simulink model "GalvoModel_v3_tfCCneu_frd"  (R2013a)
settings: Solver=ode45  StartTime=0.0  StopTime=1.5  RelTol=1e-3
values from neighbouring files (symbols this model uses):
  BEM = 108e-6    (= 0.000108)    [GalvoModel_WOK_step.m]
  CL = 180e-6    (= 0.00018)    [GalvoModel_WOK_step.m]    (also in GalvoModel_v4_sys.m = @(x,n) repmat(x, 1, n); GalvoModel_v6_sys.m = @(x,n) repmat(x, 1, n))
  CR = 2.79    [GalvoModel_WOK_step.m]
  FR = 4e-12    [GalvoModel_WOK_step.m]
  H = 0.1403    [GalvoModel_v3_discret_proc.m]
  KTR = 47e-3    (= 0.047)    [GalvoModel_WOK_step.m]
  RIN = 1.25e-8    (= 1.25e-08)    [GalvoModel_WOK_step.m]
  TRC = 6.17e-3    (= 0.00617)    [GalvoModel_WOK_step.m]
libraries: cstblocks x1
settings Model: Creator=mainster  LastModifiedBy=mainster
settings DebuggingCC: SolverPrmCheckMsg=none

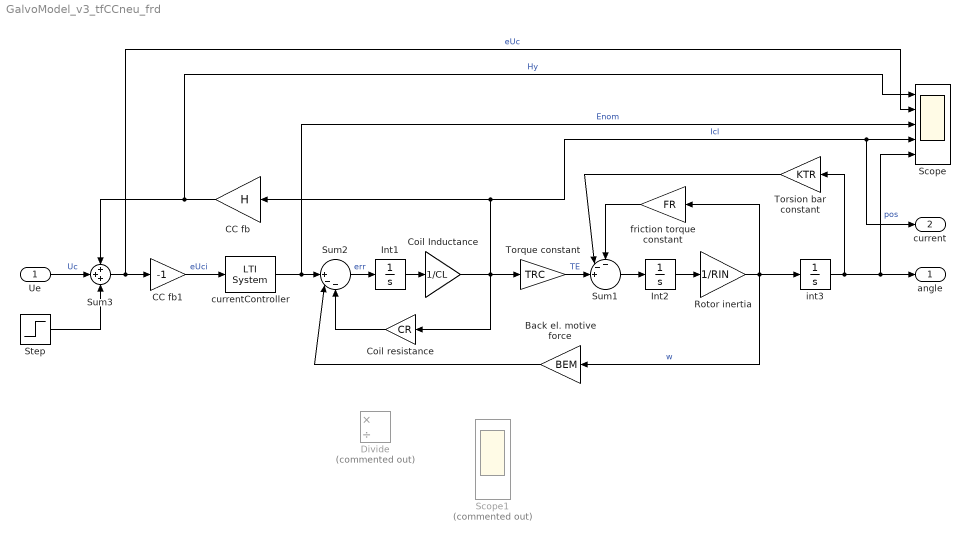
== system GalvoModel_v3_tfCCneu_frd ==
  Ue : Inport
  Back el. motive force : Gain  Gain=BEM
  CC fb : Gain  StartFcn=|  Gain=H
      | %H=100;                       
      | sprintf('StartFcn: H is %i',H)
      settings: AttributesFormatString=H=eval(%<Gain>)
  CC fb1 : Gain  StartFcn=|  Gain=-1
      | %H=100;                       
      | sprintf('StartFcn: H is %i',H)
  Coil Inductance : Gain  Gain=1/CL
  Coil resistance : Gain  Gain=CR
  Divide : Product  Commented=on  Inputs=*/
  Int1 : Integrator
  Int2 : Integrator
  Rotor inertia : Gain  Gain=1/RIN
  Scope : Scope  NumInputPorts=5
      settings: ShowLegends=on  TimeRange=1.5  YMin=-1~0.8~-15~-1~-0.2  YMax=1~1.05~5~4~1  MaxDataPoints=500000
  Scope1 : Scope  Commented=on  NumInputPorts=5
      settings: ShowLegends=on  TimeRange=1.5  YMin=-1~0.8~-15~-1~-0.2  YMax=1~1.05~5~4~1  MaxDataPoints=500000
  Step : Step  Time=0  SampleTime=0
  Sum1 : Sum  Inputs=--+||
  Sum2 : Sum  Inputs=||+--
  Sum3 : Sum  Inputs=+++
  Torque constant : Gain  Gain=TRC
  Torsion bar constant : Gain  Gain=KTR
  currentController : cstblocks/LTI System  sys=C  IC=[]
  friction torque constant : Gain  Gain=FR
  int3 : Integrator
  angle : Outport
  current : Outport  Port=2
  wires:
  Sum2/1 -> Int1/1  "err"
  Rotor inertia/1 -> Back el. motive force/1, int3/1, friction torque constant/1  "w"
  int3/1 -> Torsion bar constant/1, Scope/5, angle/1  "pos"
  Int1/1 -> Coil Inductance/1
  Coil resistance/1 -> Sum2/3
  Int2/1 -> Rotor inertia/1
  friction torque constant/1 -> Sum1/1
  Torsion bar constant/1 -> Sum1/2
  Torque constant/1 -> Sum1/3  "TE"
  Sum1/1 -> Int2/1
  Sum3/1 -> CC fb1/1, Scope/2  "eUc"
  currentController/1 -> Scope/3, Sum2/1  "Enom"
  Ue/1 -> Sum3/2  "Uc"
  Back el. motive force/1 -> Sum2/2
  Step/1 -> Sum3/3
  Coil Inductance/1 -> current/1, Scope/4, CC fb/1, Coil resistance/1, Torque constant/1  "Icl"
  CC fb/1 -> Scope/1, Sum3/1  "Hy"
  CC fb1/1 -> currentController/1  "eUci"
